simulink model "bpsk"  (R2018a)
settings: Solver=VariableStepAuto  StartTime=0.0  StopTime=0.1  RelTol=1e-3
libraries: dsparch4 x1, commrandsrc3 x1
settings Model: Creator=Administrator  LastModifiedBy=Administrator

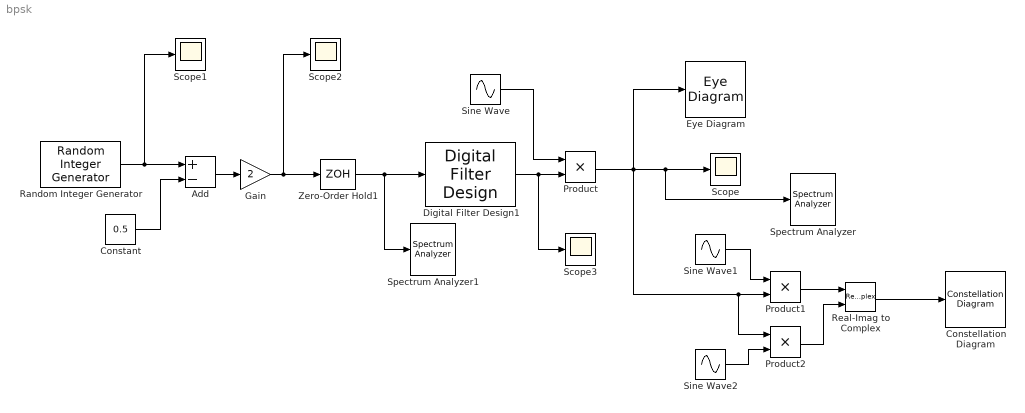
== system bpsk ==
  Add : Sum  Inputs=+-
  Constant : Constant  Value=0.5
  Constellation Diagram : ConstellationDiagram
  Digital Filter Design1 : dsparch4/Digital Filter Design  mwdsp_browser_bugfix_var=off
  Eye Diagram : EyeDiagram
  Gain : Gain  Gain=2
  Product : Product
  Product1 : Product
  Product2 : Product
  Random Integer Generator : commrandsrc3/Random Integer Generator  SetSize=2  SeedSource=Parameter  Seed=65  SampleTime=1/1e6  SamplesPerFrame=1  OutputDataType=double  SimulateUsing=Interpreted execution
  Real-Imag to Complex : RealImagToComplex
  Scope{,1..3} (4 alike) : Scope
  Sine Wave : Sin  Frequency=2*pi*1e7  Phase=pi/2  SampleTime=1/5e7
  Sine Wave1 : Sin  Frequency=2*pi*1e7  Phase=pi/2  SampleTime=1/5e7
  Sine Wave2 : Sin  Frequency=2*pi*1e7  SampleTime=1/5e7
  Spectrum Analyzer : SpectrumAnalyzer
  Spectrum Analyzer1 : SpectrumAnalyzer
  Zero-Order Hold1 : ZeroOrderHold  SampleTime=1/5e7
  wires:
  Random Integer Generator/1 -> Scope1/1, Add/1
  Constant/1 -> Add/2
  Add/1 -> Gain/1
  Product/1 -> Product2/1, Product1/2, Eye Diagram/1, Scope/1, Spectrum Analyzer/1
  Sine Wave/1 -> Product/1
  Gain/1 -> Scope2/1, Zero-Order Hold1/1
  Zero-Order Hold1/1 -> Digital Filter Design1/1, Spectrum Analyzer1/1
  Digital Filter Design1/1 -> Scope3/1, Product/2
  Sine Wave1/1 -> Product1/1
  Sine Wave2/1 -> Product2/2
  Product1/1 -> Real-Imag to Complex/1
  Product2/1 -> Real-Imag to Complex/2
  Real-Imag to Complex/1 -> Constellation Diagram/1
